simulink model "Demo1_P1C1"  (R2025b)
settings: Solver=VariableStepAuto  StartTime=0.0  StopTime=3  RelTol=1e-3
settings Model: Creator=abadirwahba  LastModifiedBy=abadirwahba

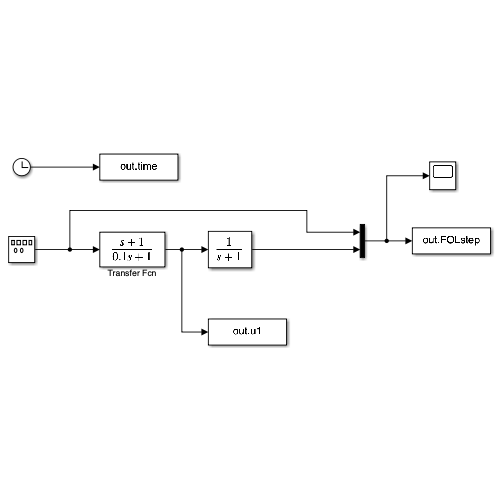
[thumbnail: Simulink's stored preview of the top-level diagram]
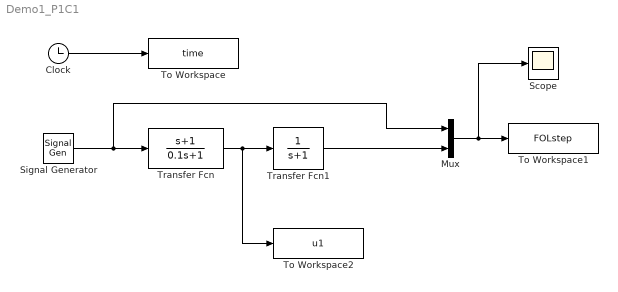
== system Demo1_P1C1 ==
  Clock : Clock
  Mux : Mux  Inputs=2
  Scope : Scope
      settings: ActiveDisplayYMinimum=-1  ActiveDisplayYMaximum=1
  Signal Generator : SignalGenerator  WaveForm=square  Frequency=0.5
  To Workspace : ToWorkspace  VariableName=time  SampleTime=-1
  To Workspace1 : ToWorkspace  VariableName=FOLstep  SampleTime=-1
  To Workspace2 : ToWorkspace  VariableName=u1  SampleTime=-1
  Transfer Fcn : TransferFcn  Numerator=[1,1]  Denominator=[0.1 1]
  Transfer Fcn1 : TransferFcn  Denominator=[1 1]
  wires:
  Clock/1 -> To Workspace/1
  Transfer Fcn/1 -> Transfer Fcn1/1, To Workspace2/1
  Transfer Fcn1/1 -> Mux/2
  Signal Generator/1 -> Mux/1, Transfer Fcn/1
  Mux/1 -> Scope/1, To Workspace1/1
